simulink subsystem "tehrani_alv_mass_balance v1"  (R2019b)
settings: Solver=VariableStepAuto  StartTime=0.0  StopTime=10.0  RelTol=1e-3
settings Model: Creator=RH  LastModifiedBy=RH

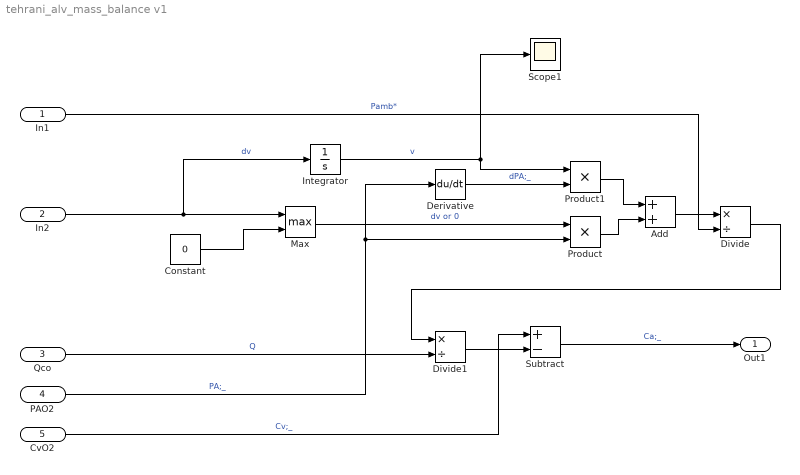
== system tehrani_alv_mass_balance v1 ==
  In1 : Inport
  In2 : Inport  Port=2
  Qco : Inport  Port=3
  PAO2 : Inport  Port=4
  CvO2 : Inport  Port=5
  Add : Sum
  Constant : Constant  Value=0
  Derivative : Derivative
  Divide : Product  Inputs=*/
  Divide1 : Product  Inputs=*/
  Integrator : Integrator
  Max : MinMax  Function=max  Inputs=2
  Product : Product
  Product1 : Product
  Scope1 : Scope
  Subtract : Sum  Inputs=+-
  Out1 : Outport
  wires:
  CvO2/1 -> Subtract/1  "Cv;_"
  Subtract/1 -> Out1/1  "Ca;_"
  Qco/1 -> Divide1/2  "Q"
  In1/1 -> Divide/2  "Pamb*"
  Product1/1 -> Add/1
  Max/1 -> Product/1  "dv or 0"
  Add/1 -> Divide/1
  Derivative/1 -> Product1/2  "dPA;_"
  Constant/1 -> Max/2
  Divide1/1 -> Subtract/2
  In2/1 -> Max/1, Integrator/1  "dv"
  PAO2/1 -> Derivative/1, Product/2  "PA;_"
  Integrator/1 -> Product1/1, Scope1/1  "v"
  Divide/1 -> Divide1/1
  Product/1 -> Add/2
